simulink model "test"  (R2022a)
settings: Solver=VariableStepAuto  StartTime=0.0  StopTime=380  RelTol=1e-3
values from neighbouring files (symbols this model uses):
  acc_sigmax = 2.6e-3    (= 0.0026)    [init.m]
  acc_sigmay = 2.6e-3    (= 0.0026)    [init.m]
  acc_sigmaz = 2.6e-3    (= 0.0026)    [init.m]
  bias_hat_0 = [gyro_biasx + bias_eps_x; gyro_biasy + bias_eps_y; gyro_biasz + bias_eps_z]    [init.m]
  EN_OUTAGE = true    [init.m]
  g = [0; 0; 9.81]    [init.m]
  gps_sigmax = 3    [init.m]
  gps_sigmay = 3    [init.m]
  gps_sigmaz = 3    [init.m]
  gyro_biasx = deg2rad(.05)    [init.m]
  gyro_biasy = 2*deg2rad(.05)    [init.m]
  gyro_biasz = 3*deg2rad(.05)    [init.m]
  gyro_sigmax = deg2rad(0.18)    [init.m]
  gyro_sigmay = deg2rad(0.18)    [init.m]
  gyro_sigmaz = deg2rad(0.18)    [init.m]
  interval1 = [100; 140]    [init.m]
  interval2 = [280; 320]    [init.m]
  K1_lambda = K_inf(1:3,:)    [gain_lambda.m]
  K1_p = K_inf(1:3,:)    [gain_p.m]    (also in init.m = 0.59*eye(3))
  K2_lambda = K_inf(4:6,:)    [gain_lambda.m]
  K2_p = K_inf(4:6,:)    [gain_p.m]    (also in init.m = 0.14*eye(3))
  lambda0 = [0;0;0]    [init.m]
  lambda_hat_0 = [0;0;0]    [init.m]
  m = [270; 100; 0]    [init.m]
  mag_sigmax = 1    [init.m]
  mag_sigmay = 1    [init.m]
  mag_sigmaz = 1    [init.m]
  p_hat_0 = [0;0;0]    [init.m]
  T = 1/56    (= 0.0178571428571)    [frequency_analysi.m]    (also in init.m)
  T_gps = 14*T    [gain_p.m]    (also in init.m = 0.25)
  v_B_hat_0 = [0; 0; 0]    [init.m]
undefined symbols (not defined in the file or in its folder): sigbuilder_block
libraries: matrix_library x1
settings Model: Creator=morel  LastModifiedBy=Leo
settings ModelReferenceCC: EnableRefExpFcnMdlSchedulingChecks=off
settings RTWCC: Description=Generic Real-Time Target

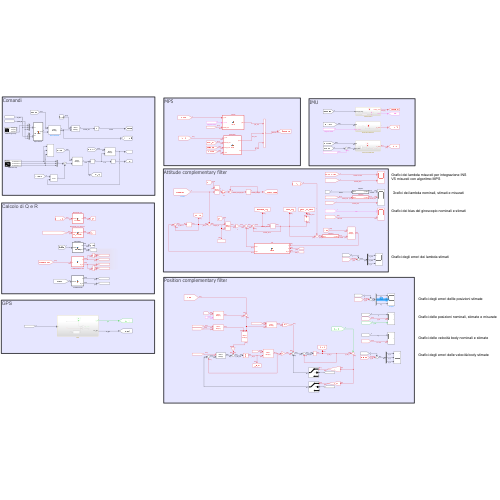
[thumbnail: Simulink's stored preview of the top-level diagram]
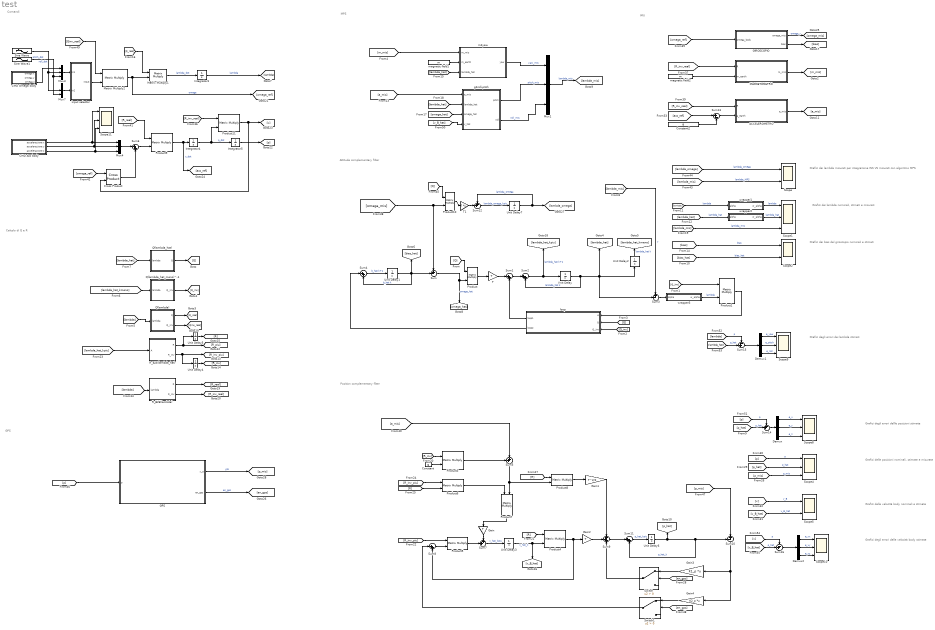
== system test ==
  note: Grafici dei lambda misurati per integrazione INS VS misurati con algoritmo MPS
  note: GPS
  note: Calcolo di Q e R
  note: IMU
  note: Comandi
  note: Position complementary filter
  note: MPS
  note: Attitude complementary filter
  note: Grafici dei lambda nominali, stimati e misurati
  note: Grafici dei bias del giroscopio nominali e stimati
  note: Grafici degli errori dei lambda stimati
  note: Grafici degli errori dellle posizioni stimate
  note: Grafici delle posizioni nominali, stimate e misurate
  note: Grafici delle velocità body nominali e stimate
  note: Grafici degli errori delle velocità body stimate
  ACCELEROMETRO : Subsystem
  CMD Acc body : Subsystem  Tag=STV Subsys  LoadFcn=sigbuilder_block('load',[182.4 90 550.8 320.4 ]);  StartFcn=sigbuilder_block('start');  StopFcn=sigbuilder_block('stop');  ClipboardFcn=sigbuilder_block('clipboard');  mask(Sigbuilder block){tuvar=[0:10]}
      mask help: Simulink:masks:SigbuilderBlock_MD
      mask init:
      | if ~strcmp(get_param(bdroot(gcbh),'SimulationStatus'),'stopped') tuvar = sigbuilder_block('maskInit'); end
      settings: CopyFcn=sigbuilder_block('copy');  DeleteFcn=sigbuilder_block('delete');  ModelCloseFcn=sigbuilder_block('modelClose');  PreSaveFcn=sigbuilder_block('preSave');  PauseFcn=sigbuilder_block('pause');  ContinueFcn=sigbuilder_block('continue');  NameChangeFcn=sigbuilder_block('namechange');  OpenFcn=sigbuilder_block('open',[182.4 90 550.8 320.4 ]);  CloseFcn=sigbuilder_block('close');
      mask Display: plot(0, 0, 100, 100,[2, 2, 32, 32, 2], [68, 8, 8, 68, 68],[32, 2], [38, 38], [32, 19, 2],[53, 60, 44], [32, 17, 17, 2],[16, 16, 31, 31]);txt = getActiveGroup(gcbh);text(2, 100, txt,'verticalAlignment', 'top');
  CMD Omega body : Subsystem  Tag=STV Subsys  LoadFcn=sigbuilder_block('load');  StartFcn=sigbuilder_block('start');  StopFcn=sigbuilder_block('stop');  ClipboardFcn=sigbuilder_block('clipboard');  mask(Sigbuilder block){tuvar=[0:10]}
      mask help: Simulink:masks:SigbuilderBlock_MD
      mask init:
      | if ~strcmp(get_param(bdroot(gcbh),'SimulationStatus'),'stopped') tuvar = sigbuilder_block('maskInit'); end
      settings: CopyFcn=sigbuilder_block('copy');  DeleteFcn=sigbuilder_block('delete');  ModelCloseFcn=sigbuilder_block('modelClose');  PreSaveFcn=sigbuilder_block('preSave');  PauseFcn=sigbuilder_block('pause');  ContinueFcn=sigbuilder_block('continue');  NameChangeFcn=sigbuilder_block('namechange');  OpenFcn=sigbuilder_block('open',[112.8 93.6 550.8 400.2 ]);  CloseFcn=sigbuilder_block('close');
      mask Display: plot(0, 0, 100, 100,[2, 2, 32, 32, 2], [68, 8, 8, 68, 68],[32, 2], [38, 38], [32, 19, 2],[53, 60, 44], [32, 17, 17, 2],[16, 16, 31, 31]);txt = getActiveGroup(gcbh);text(2, 100, txt,'verticalAlignment', 'top');
  Constant : Constant  Value=g  VectorParams1D=off
  Constant2 : Constant  Value=g  VectorParams1D=off
  Cross Product : matrix_library/Cross Product
      settings: SourceProductBaseCode=SL
  Demux : Demux  Outputs=3
  Demux1 : Demux  Outputs=3
  Demux2 : Demux  Outputs=3
  GIROSCOPIO : Subsystem
  GPS : Subsystem
  Gain : Gain  Gain=T
  Gain1 : Gain  Gain=T^2/2
  Gain2 : Gain  Gain=T
  Gain3 : Gain  Gain=K1_p  Multiplication=Matrix(K*u)
  Gain4 : Gain  Gain=K2_p  Multiplication=Matrix(K*u)
  Integrator3 : Integrator  InitialCondition=lambda0
  Integrator4 : Integrator  InitialCondition=[0;0;0]
  Integrator5 : Integrator
  MAGNETOMETRO : Subsystem
  Matrix Multiply1 : Product  Multiplication=Matrix(*)
  Matrix Multiply2 : Product  Multiplication=Matrix(*)
  Mux{1,3..4,7} (4 alike) : Mux  Inputs=3
  Product{,1,3..11} (11 alike) : Product  Multiplication=Matrix(*)
  Q(lambda) : MATLAB Function  TreatAsAtomicUnit=on
  Q(lambda_hat) : MATLAB Function  TreatAsAtomicUnit=on
  Q(lambda_hat_meno)^-1 : MATLAB Function  TreatAsAtomicUnit=on
  R_B2E(lambda) : MATLAB Function  TreatAsAtomicUnit=on
  R_B2E(lambda_hat) : MATLAB Function  TreatAsAtomicUnit=on
  Scope : Scope  NumInputPorts=2
  Scope{1,4,8..11} (6 alike) : Scope  NumInputPorts=3
  Scope2 : Scope  NumInputPorts=2
  Scope5 : Scope  NumInputPorts=2
  Sine Wave : Sin  Amplitude=deg2rad(10)*(2*pi*0.01)  Frequency=2*pi*0.01  SampleTime=0
  Sine Wave1 : Sin  Amplitude=deg2rad(9)*(2*pi*0.01)  Frequency=2*pi*0.01  Phase=2  SampleTime=0
  Sum : Sum  Inputs=+-|
  Sum{1..2,4,6,8,11} (6 alike) : Sum  Inputs=|++
  Sum{10,14..16} (4 alike) : Sum  Inputs=-+|
  Sum12 : Sum  Inputs=++|
  Sum13 : Sum  Inputs=|+-
  Sum3 : Sum  Inputs=+-|
  Sum5 : Sum  Inputs=++|
  Sum7 : Sum  Inputs=++|
  Sum9 : Sum  Inputs=+++
  Switch : Switch  Criteria=u2 > Threshold  SaturateOnIntegerOverflow=off  InputSameDT=off
  Switch1 : Switch  Criteria=u2 > Threshold  SaturateOnIntegerOverflow=off  InputSameDT=off
  T : Gain  Gain=T
  T1 : Gain  Gain=T  Multiplication=Matrix(K*u)
  Unit Delay : UnitDelay  InitialCondition=lambda_hat_0  SampleTime=T  HasFrameUpgradeWarning=on
  Unit Delay1 : UnitDelay  InitialCondition=bias_hat_0  SampleTime=T  HasFrameUpgradeWarning=on
  Unit Delay2 : UnitDelay  InitialCondition=lambda_hat_0  SampleTime=T  HasFrameUpgradeWarning=on
  Unit Delay3 : UnitDelay  InitialCondition=v_B_hat_0  SampleTime=-1  HasFrameUpgradeWarning=on
  Unit Delay4 : UnitDelay  SampleTime=T  HasFrameUpgradeWarning=on
  Unit Delay5 : UnitDelay  SampleTime=T  HasFrameUpgradeWarning=on
  Unit Delay6 : UnitDelay  InitialCondition=p_hat_0  SampleTime=-1  HasFrameUpgradeWarning=on
  Unit Delay7 : UnitDelay  InitialCondition=lambda_hat_0  SampleTime=T  HasFrameUpgradeWarning=on
  g2roll-pitch : MATLAB Function  TreatAsAtomicUnit=on
  input selector : MATLAB Function  TreatAsAtomicUnit=on
  loop : MATLAB Function  TreatAsAtomicUnit=on
  m2yaw : MATLAB Function  TreatAsAtomicUnit=on
  magnetic field1 : Constant  Value=m
  magnetic field2 : Constant  Value=m
  wrapper1 : MATLAB Function  TreatAsAtomicUnit=on
  wrapper2 : MATLAB Function  TreatAsAtomicUnit=on
  wrapper3 : MATLAB Function  TreatAsAtomicUnit=on
  wires:
  Sum/1 -> [omega_hat], Product/2  "omega_hat"
  Q(lambda_hat)/1(Q) -> [Q]
  Product/1 -> T/1
  T/1 -> Sum1/1
  Sum1/1 -> Sum2/1
  Sum2/1 -> [lambda_hat_kpiu], Unit Delay/1  "lambda_hat k+1"
  Unit Delay/1 -> Sum2/2, Sum3/2, [lambda_hat], Unit Delay2/1  "lambda_hat k"
  Product1/1 -> loop/1(e)
  [Q] -> Product/1
  Q(lambda_hat_meno)^-1/1(Q_inv) -> [Q_inv]
  loop/1(loop1) -> Sum1/2
  loop/2(loop2) -> Sum4/1
  Sum4/1 -> Unit Delay1/1  "b_hat k+1"
  Unit Delay1/1 -> Sum/2, Sum4/2, [bias_hat]  "b_hat k"
  [Q] -> loop/2(Q)
  [Q_inv] -> loop/3(Q_inv)
  Q(lambda)/1(Q) -> [Q_real]
  [lambda] -> Q(lambda)/1(lambda)
  [lambda_hat_kmeno] -> Q(lambda_hat_meno)^-1/1(lambda)
  [lambda_hat] -> Q(lambda_hat)/1(lambda)
  [Q_inv] -> Product1/1
  Unit Delay2/1 -> [lambda_hat_kmeno]  "lambda_hat k"
  [lambda_mis] -> Sum3/1  "y"
  [lambda] -> wrapper1/1(alpha)  "lambda"
  [lambda_hat] -> wrapper2/1(alpha)  "lambda_hat"
  [bias] -> Scope2/1  "bias"
  [bias_hat] -> Scope2/2  "bias_hat"
  [lambda_hat] -> m2yaw/3(lambda_hat)
  magnetic field1/1 -> m2yaw/2(m_earth)
  [lambda_hat] -> g2roll-pitch/2(lambda_hat)
  [m_mis] -> m2yaw/1(m_mis)
  [a_mis] -> g2roll-pitch/1(a_mis)
  m2yaw/1(yaw) -> Mux1/1  "yaw_mis"
  g2roll-pitch/1(pitch) -> Mux1/2  "pitch_mis"
  g2roll-pitch/2(roll) -> Mux1/3  "roll_mis"
  [omega_hat] -> g2roll-pitch/3(omega_hat)
  Mux1/1 -> [lambda_mis]  "lambda_mis"
  [lambda_mis] -> Scope1/3  "lambda_mis"
  Gain1/1 -> Sum9/1
  [R_inv_piu] -> Product6/1
  Product6/1 -> Product7/1
  [R] -> Product8/1
  Product7/1 -> Gain/1
  [R_inv_piu] -> Product5/1
  Product8/1 -> Gain1/1
  Gain3/1 -> Switch/1
  Sum10/1 -> Gain4/1, Gain3/1
  Sum9/1 -> Sum11/1
  Unit Delay5/1 -> [R]
  [lambda_hat_kpiu] -> R_B2E(lambda_hat)/1(A)
  Unit Delay6/1 -> Sum10/1, Sum11/2, [p_hat]  "p_hat_k"
  [R] -> Product4/1
  [R] -> Product6/2
  Unit Delay4/1 -> [R_inv]
  Unit Delay3/1 -> [v_B_hat], Product4/2  "v_hat_k"
  Product5/1 -> Sum7/2
  Sum7/1 -> Unit Delay3/1  "v_hat_kpiu"
  Sum8/1 -> Product5/2
  Switch1/1 -> Sum8/1
  Sum5/1 -> Product7/2, Product8/2
  Gain/1 -> Sum7/1
  Sum11/1 -> Unit Delay6/1  "p_hat_kpiu"
  Gain2/1 -> Sum9/2
  R_B2E(lambda_hat)/1(R) -> Unit Delay5/1, [R_piu]
  [R_inv] -> Product3/1
  Product3/1 -> Sum5/1
  Product4/1 -> Gain2/1, Sum8/2
  R_B2E(lambda_hat)/2(R_inv) -> [R_inv_piu], Unit Delay4/1
  Constant/1 -> Product3/2
  [p] -> Scope4/1  "p"
  [p_hat] -> Scope4/2  "p_hat"
  [v_B_hat] -> Scope5/2  "v_B_hat"
  [v] -> Scope5/1  "v_B"
  R_B2E(lambda)/1(R) -> [R_real]
  R_B2E(lambda)/2(R_inv) -> [R_inv_real]
  [lambda] -> R_B2E(lambda)/1(lambda)
  [Q_real] -> Matrix Multiply1/1
  Matrix Multiply1/1 -> Integrator3/1  "lambda_dot"
  Mux3/1 -> input selector/1(in1)
  [R_inv_real] -> Product11/1
  Product9/1 -> [acc_ref], Integrator4/1  "v_dot"
  Integrator4/1 -> Product11/2, Integrator5/1  "p_dot"
  Integrator5/1 -> [p]
  Product11/1 -> Cross Product/2, [v]
  CMD Acc body/1(accelerazione x) -> Scope11/1, Mux4/1
  CMD Acc body/2(accelerazione y) -> Scope11/2, Mux4/2
  CMD Acc body/3(accelerazione z) -> Mux4/3, Scope11/3
  [omega_ref] -> GIROSCOPIO/1(omega_body)
  [R_inv_real] -> MAGNETOMETRO/1(R)
  magnetic field2/1 -> MAGNETOMETRO/2(m_earth)
  GIROSCOPIO/1(omega_mis) -> [omega_mis]  "omega_r"
  [omega_mis] -> Product10/2, Sum/1
  MAGNETOMETRO/1(m_mis) -> [m_mis]
  [acc_ref] -> Sum13/1
  Sum13/1 -> ACCELEROMETRO/2(a_earth)
  [R_inv_real] -> ACCELEROMETRO/1(R)
  Constant2/1 -> Sum13/2
  ACCELEROMETRO/1(a_mis) -> [a_mis]
  [a_mis] -> Sum5/2
  Integrator3/1 -> [lambda]  "lambda"
  GIROSCOPIO/2(bias) -> [bias]
  [p_mis] -> Scope4/3  "p_mis"
  Mux4/1 -> Sum6/1
  [R_real] -> Product9/1
  Sum6/1 -> Product9/2
  [omega_ref] -> Cross Product/1
  Cross Product/1 -> Sum6/2
  [lambda_mis] -> Scope/2  "lambda_MPS"
  Unit Delay7/1 -> [lambda_omega], Sum12/1  "lambda_omega"
  Sum12/1 -> Unit Delay7/1  "lambda_omega_kpiu"
  [lambda_omega] -> Scope/1  "lambda_omega"
  T1/1 -> Sum12/2
  [Q] -> Product10/1
  Product10/1 -> T1/1
  GPS/1(y_p) -> [p_mis]  "ypk"
  [p] -> GPS/1(p)
  [p_mis] -> Sum10/2
  GPS/2(en_gps) -> [en_gps]  "en_gps"
  Switch/1 -> Sum9/3
  Gain4/1 -> Switch1/1
  [en_gps] -> Switch/2
  [en_gps] -> Switch1/2
  Sine Wave1/1 -> Mux7/3, Mux3/3  "pitch_dot"
  Sine Wave/1 -> Mux7/2, Mux3/2  "roll_dot"
  [Qinv_real] -> Matrix Multiply2/1
  Matrix Multiply2/1 -> [omega_ref], Matrix Multiply1/2  "omega"
  Q(lambda)/2(Q_inv) -> [Qinv_real]
  CMD Omega body/3(omega z) -> Mux3/1
  [v_B_hat] -> g2roll-pitch/4(v_hat)
  wrapper1/1(w_alpha) -> Scope1/1  "lambda"
  Sum3/1 -> wrapper3/1(alpha)
  wrapper3/1(w_alpha) -> Product1/2  "lambda"
  wrapper2/1(w_alpha) -> Scope1/2  "lambda_hat"
  [p] -> Sum14/1  "p"
  [p_hat] -> Sum14/2  "p_hat"
  Sum14/1 -> Demux/1
  Demux/1 -> Scope8/1  "e_x"
  Demux/2 -> Scope8/2  "e_y"
  Demux/3 -> Scope8/3  "e_z"
  [lambda_hat] -> Sum15/2  "p_hat"
  Demux1/2 -> Scope9/2  "e_pitch"
  Demux1/3 -> Scope9/3  "e_roll"
  Demux1/1 -> Scope9/1  "e_yaw"
  [lambda] -> Sum15/1  "p"
  Sum15/1 -> Demux1/1
  [v_B_hat] -> Sum16/2  "p_hat"
  Demux2/2 -> Scope10/2  "e_vy"
  Demux2/3 -> Scope10/3  "e_vz"
  Demux2/1 -> Scope10/1  "e_vx"
  [v] -> Sum16/1  "p"
  Sum16/1 -> Demux2/1
  Mux7/1 -> input selector/2(in2)
  input selector/1(input) -> Matrix Multiply2/2

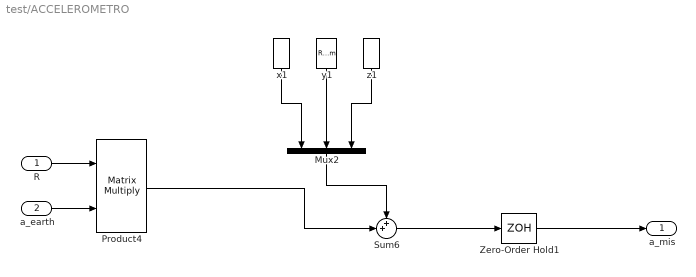
== system test/ACCELEROMETRO ==
  R : Inport
  a_earth : Inport  Port=2
  Mux2 : Mux  Inputs=3
  Product4 : Product  Multiplication=Matrix(*)
  Sum6 : Sum  Inputs=++|
  Zero-Order Hold1 : ZeroOrderHold  SampleTime=T
  x1 : RandomNumber  Variance=acc_sigmax  SampleTime=T
  y1 : RandomNumber  Variance=acc_sigmay  SampleTime=T  VectorParams1D=off
  z1 : RandomNumber  Variance=acc_sigmaz  SampleTime=T
  a_mis : Outport
  wires:
  z1/1 -> Mux2/3
  x1/1 -> Mux2/1
  y1/1 -> Mux2/2
  R/1 -> Product4/1
  Mux2/1 -> Sum6/1
  a_earth/1 -> Product4/2
  Sum6/1 -> Zero-Order Hold1/1
  Product4/1 -> Sum6/2
  Zero-Order Hold1/1 -> a_mis/1

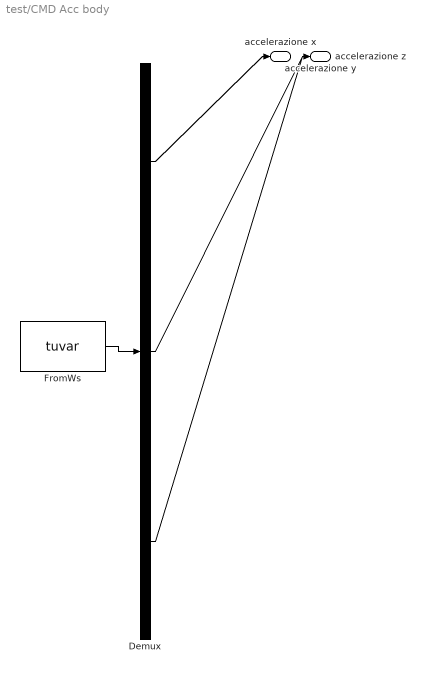
== system test/CMD Acc body ==
  Demux : Demux  Tag=STV Demux  Outputs=3
      settings: DisplayOption=none
  FromWs : FromWorkspace  Tag=STV FromWs  VariableName=tuvar
      SigBuilderData=|
      | common.afterFinalStr = 'Extrapolate'
      | common.sampleTime = 0
      | dataSet.timeRange = [0 10]
      | dataSet.name = 'Group 1'
      | sbobj.Groups.Name = 'Group 1'
      | sbobj.Groups.Signals(1).Name = 'accelerazione x'
      | sbobj.Groups.Signals(1).XData = [0 4 5 6 7.5 8.5 10]
      | sbobj.Groups.Signals(1).YData = [0 0 0.8 0 1.2 0 0]
      | sbobj.Groups.Signals(2).Name = 'accelerazione y'
      | sbobj.Groups.Signals(2).XData = [0 10]
      | sbobj.Groups.Signals(2).YData = [0 0]
      | sbobj.Groups.Signals(3).Name = 'accelerazione z'
      | sbobj.Groups.Signals(3).XData = [0 4 6 10]
      | sbobj.Groups.Signals(3).YData = [0 0 0 0]
  accelerazione x : Outport  Tag=STV Outport
  accelerazione y : Outport  Tag=STV Outport  Port=2
  accelerazione z : Outport  Tag=STV Outport  Port=3
  wires:
  FromWs/1 -> Demux/1
  Demux/1 -> accelerazione x/1
  Demux/2 -> accelerazione y/1
  Demux/3 -> accelerazione z/1

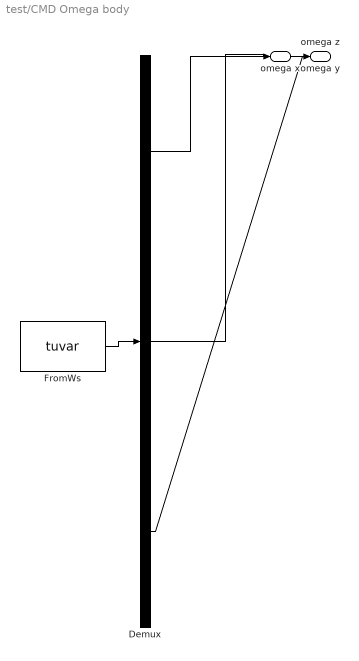
== system test/CMD Omega body ==
  Demux : Demux  Tag=STV Demux  Outputs=3
      settings: DisplayOption=none
  FromWs : FromWorkspace  Tag=STV FromWs  VariableName=tuvar
      SigBuilderData=|
      | common.afterFinalStr = 'Extrapolate'
      | common.sampleTime = 0
      | dataSet.timeRange = [0 10]
      | dataSet.name = 'Group 1'
      | sbobj.Groups.Name = 'Group 1'
      | sbobj.Groups.Signals(1).Name = 'omega x'
      | sbobj.Groups.Signals(1).XData = [0 4 6 10]
      | sbobj.Groups.Signals(1).YData = [0 0 0 0]
      | sbobj.Groups.Signals(2).Name = 'omega y'
      | sbobj.Groups.Signals(2).XData = [0 2.02 3.02 4.96 10]
      | sbobj.Groups.Signals(2).YData = [0 0 0.3 0 0]
      | sbobj.Groups.Signals(3).Name = 'omega z'
      | sbobj.Groups.Signals(3).XData = [0 4 6 10]
      | sbobj.Groups.Signals(3).YData = [0.05 0.05 0.05 0.05]
  omega x : Outport  Tag=STV Outport
  omega y : Outport  Tag=STV Outport  Port=2
  omega z : Outport  Tag=STV Outport  Port=3
  wires:
  Demux/1 -> omega x/1
  FromWs/1 -> Demux/1
  Demux/2 -> omega y/1
  Demux/3 -> omega z/1

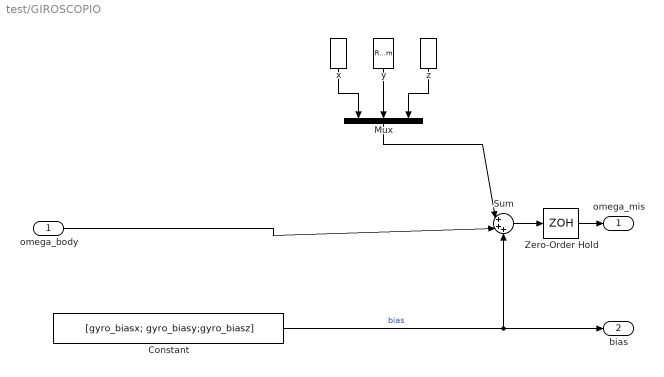
== system test/GIROSCOPIO ==
  omega_body : Inport
  Constant : Constant  Value=[gyro_biasx; gyro_biasy;gyro_biasz]
  Mux : Mux  Inputs=3
  Sum : Sum  Inputs=|+++
  Zero-Order Hold : ZeroOrderHold  SampleTime=T
  x : RandomNumber  Variance=gyro_sigmax  SampleTime=T
  y : RandomNumber  Variance=gyro_sigmay  SampleTime=T  VectorParams1D=off
  z : RandomNumber  Variance=gyro_sigmaz  SampleTime=T
  omega_mis : Outport
  bias : Outport  Port=2
  wires:
  omega_body/1 -> Sum/2
  Sum/1 -> Zero-Order Hold/1
  y/1 -> Mux/2
  x/1 -> Mux/1
  z/1 -> Mux/3
  Mux/1 -> Sum/1
  Zero-Order Hold/1 -> omega_mis/1
  Constant/1 -> bias/1, Sum/3  "bias"

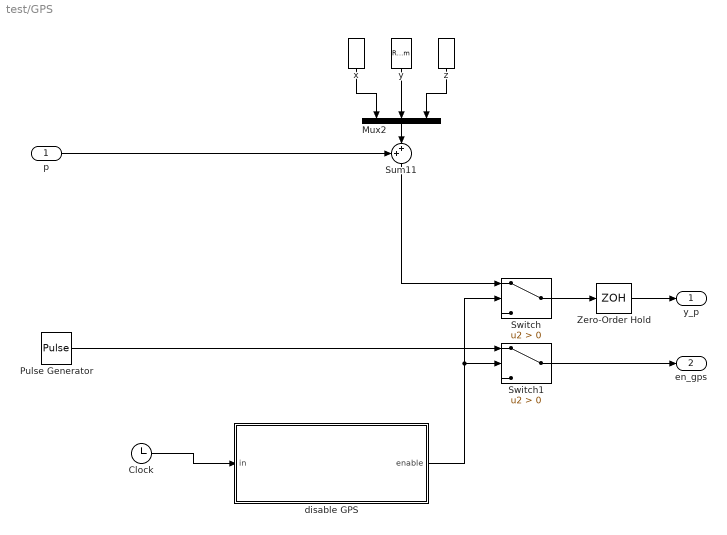
== system test/GPS ==
  p : Inport
  Clock : Clock
  Mux2 : Mux  Inputs=3
  Pulse Generator : DiscretePulseGenerator  PulseType=Time based  Period=T_gps  PulseWidth=5
  Sum11 : Sum  Inputs=++|
  Switch : Switch  Criteria=u2 > Threshold  SaturateOnIntegerOverflow=off  InputSameDT=off
  Switch1 : Switch  Criteria=u2 > Threshold  SaturateOnIntegerOverflow=off  InputSameDT=off
  Zero-Order Hold : ZeroOrderHold  SampleTime=T_gps
  disable GPS : MATLAB Function  TreatAsAtomicUnit=on
  x : RandomNumber  Variance=gps_sigmax  SampleTime=T_gps
  y : RandomNumber  Variance=gps_sigmay  SampleTime=T_gps  VectorParams1D=off
  z : RandomNumber  Variance=gps_sigmaz  SampleTime=T_gps
  y_p : Outport
  en_gps : Outport  Port=2
  wires:
  Mux2/1 -> Sum11/2
  z/1 -> Mux2/3
  y/1 -> Mux2/2
  x/1 -> Mux2/1
  Sum11/1 -> Switch/1
  Zero-Order Hold/1 -> y_p/1
  Pulse Generator/1 -> Switch1/1
  p/1 -> Sum11/1
  Switch1/1 -> en_gps/1
  Switch/1 -> Zero-Order Hold/1
  disable GPS/1(enable) -> Switch1/2, Switch/2
  Clock/1 -> disable GPS/1(in)

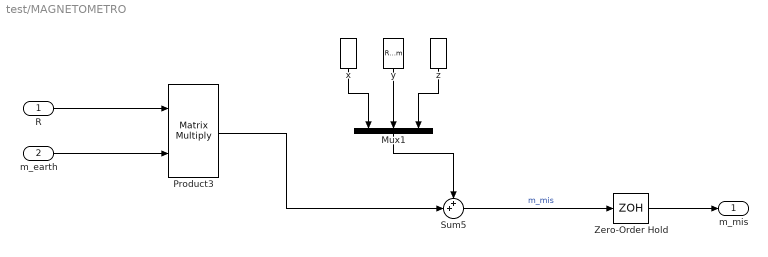
== system test/MAGNETOMETRO ==
  R : Inport
  m_earth : Inport  Port=2
  Mux1 : Mux  Inputs=3
  Product3 : Product  Multiplication=Matrix(*)
  Sum5 : Sum  Inputs=++|
  Zero-Order Hold : ZeroOrderHold  SampleTime=T
  x : RandomNumber  Variance=mag_sigmax  SampleTime=T
  y : RandomNumber  Variance=mag_sigmay  SampleTime=T  VectorParams1D=off
  z : RandomNumber  Variance=mag_sigmaz  SampleTime=T
  m_mis : Outport
  wires:
  R/1 -> Product3/1
  z/1 -> Mux1/3
  y/1 -> Mux1/2
  Product3/1 -> Sum5/2
  Mux1/1 -> Sum5/1
  x/1 -> Mux1/1
  Sum5/1 -> Zero-Order Hold/1  "m_mis"
  m_earth/1 -> Product3/2
  Zero-Order Hold/1 -> m_mis/1

== matlab function test/wrapper3 ==
  data: alpha input; w_alpha output
function w_alpha  = wtp(alpha)

w_alpha =  wrapToPi(alpha);

== matlab function test/wrapper2 ==
  data: alpha input; w_alpha output
function w_alpha  = wtp(alpha)

w_alpha =  wrapToPi(alpha);

== matlab function test/input selector ==
  data: in1 input; input output; in2 input; TRAIETTORIA parameter
function input = inputSelector(in1, in2, TRAIETTORIA)
    % inserire condizioni per cui disabilitare il GPS
    switch TRAIETTORIA
        case 1 
            input = in1;
        case 2
            input = in2;
        otherwise
            input = [0;0;0];
    end
end

== matlab function test/Q(lambda_hat_meno)^-1 ==
  settings: updateMethod=DISCRETE  sampleTime=T
  data: lambda input; Q_inv output
function Q_inv = inv_kinematic(lambda)

r = lambda(3);
p = lambda(2);


Q_inv = inv([   0 sin(r)*sec(p) cos(r)*sec(p);
        0 cos(r)        -sin(r);
        1 sin(r)*tan(p)  cos(r)*tan(p);]);

== matlab function test/Q(lambda_hat) ==
  settings: updateMethod=DISCRETE  sampleTime=T
  data: lambda input; Q output
function Q = kinematic(lambda)

r = lambda(3);
p = lambda(2);


Q = [   0 sin(r)*sec(p) cos(r)*sec(p);
        0 cos(r)        -sin(r);
        1 sin(r)*tan(p)  cos(r)*tan(p);];

== matlab function test/loop ==
  data: e input; loop1 output; Q input; Q_inv input; K1_lambda parameter; loop2 output; K2_lambda parameter
function [loop1,loop2] = Gains(e,Q,Q_inv,K1_lambda,K2_lambda)


loop1 =  (Q*(K1_lambda-eye(3))+ inv(Q_inv))*e;                 
loop2 = K2_lambda*e;

== matlab function test/Q(lambda) ==
  data: lambda input; Q output; Q_inv output
function [Q, Q_inv] = kinematic(lambda)

r = lambda(3);
p = lambda(2);


Q = [   0 sin(r)*sec(p) cos(r)*sec(p);
        0 cos(r)        -sin(r);
        1 sin(r)*tan(p)  cos(r)*tan(p);];

Q_inv =Q^(-1);

== matlab function test/g2roll-pitch ==
  data: pitch output; a_mis input; lambda_hat input; roll output; omega_hat input; v_hat input
function [pitch, roll] = a2rp(a_mis, lambda_hat, omega_hat, v_hat)
r = lambda_hat(3);

a_p = a_mis - cross(omega_hat,v_hat);

roll = atan2(-a_p(2),-a_p(3));
if cos(r)~=0
    pitch = atan(-a_p(1)*cos(r)/a_p(3));
else 
    pitch = atan(-a_p(1)*sin(r)/a_p(2));
end

== matlab function test/m2yaw ==
  data: m_mis input; m_earth input; lambda_hat input; yaw output
function yaw = m2yaw(m_mis, m_earth, lambda_hat)

r = lambda_hat(3);
p = lambda_hat(2);

Rx = [  1, 0, 0;
        0, cos(r), sin(r);
        0, -sin(r), cos(r)]';

Ry = [  cos(p), 0, -sin(p);
        0, 1, 0;
        sin(p), 0, cos(p)]';

m_proj = Ry*Rx*m_mis;

a1 = m_earth(2)*m_proj(1) - m_earth(1)*m_proj(2);
a2 = m_earth(1)*m_proj(1) + m_earth(2)*m_proj(2);
yaw = atan2(a1, a2);

== matlab function test/R_B2E(lambda_hat) ==
  data: A input; R output; R_inv output
function [R , R_inv] = rot(A)

r = A(3);
p = A(2);
y = A(1);

Rx = [  1      0        0     ;
        0    cos(r)  -sin(r)  ;
        0    sin(r)   cos(r)] ;

Ry = [  cos(p)      0        sin(p) ;
          0         1          0    ;
       -sin(p)      0        cos(p)];

Rz = [  cos(y)    -sin(y)     0 ;
        sin(y)     cos(y)     0 ;
          0           0       1];


R = Rz*Ry*Rx; 
R_inv = transpose(R);

== matlab function test/GPS/disable GPS ==
  data: in input; EN_OUTAGE parameter; enable output; interval1 parameter; interval2 parameter
function enable = disableGPS(in, EN_OUTAGE, interval1, interval2)
% inserire condizioni per cui disabilitare il GPS
if ~EN_OUTAGE 
    enable = 1;
    return;
end
if (in > interval1(1) && in < interval1(2))||(in > interval2(1) && in < interval2(2))
    enable = 0;
else
    enable = 1;
end

== matlab function test/R_B2E(lambda) ==
  data: lambda input; R output; R_inv output
function [R , R_inv] = rot(lambda)

r = lambda(3);
p = lambda(2);
y = lambda(1);

Rx = [  1      0        0     ;
        0    cos(r)  -sin(r)  ;
        0    sin(r)   cos(r)] ;

Ry = [  cos(p)      0        sin(p) ;
          0         1          0    ;
       -sin(p)      0        cos(p)];

Rz = [  cos(y)    -sin(y)     0 ;
        sin(y)     cos(y)     0 ;
          0           0       1];


R = Rz*Ry*Rx; 
R_inv = transpose(R);

== matlab function test/wrapper1 ==
  data: alpha input; w_alpha output
function w_alpha  = wtp(alpha)

w_alpha =  wrapToPi(alpha);
